simulink model "Control_pendulum_LQR"  (R2023b)
settings: Solver=VariableStepAuto  StartTime=0.0  StopTime=10.0  RelTol=1e-3
settings Model: Creator=Administrator  LastModifiedBy=Administrator

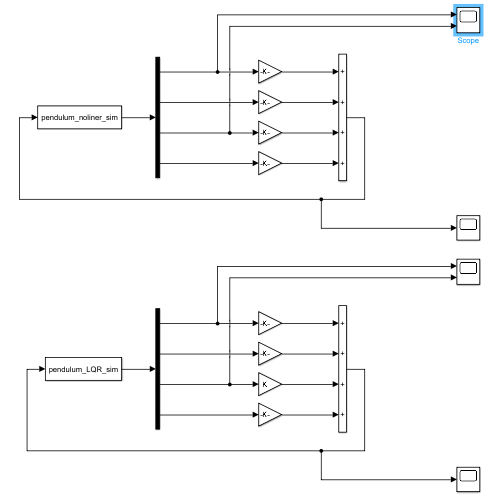
[thumbnail: Simulink's stored preview of the top-level diagram]
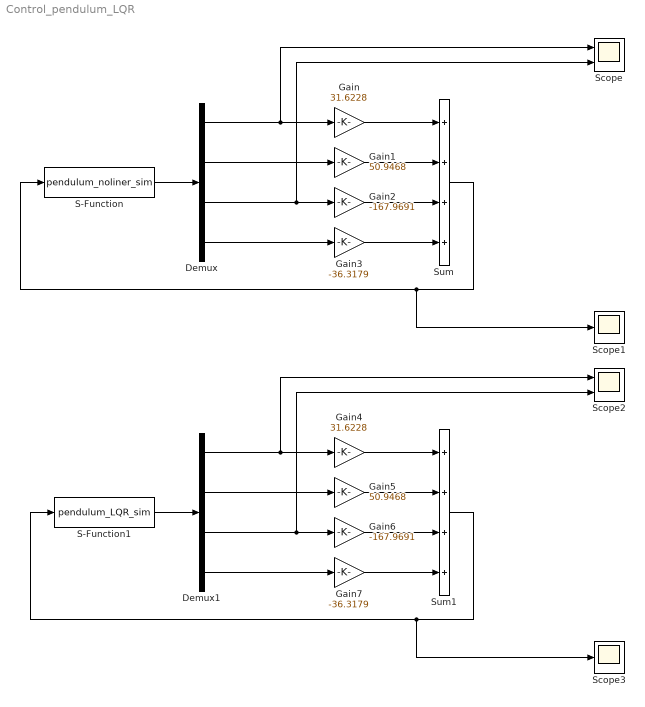
== system Control_pendulum_LQR ==
  Demux : Demux
  Demux1 : Demux
  Gain : Gain  Gain=31.6228
  Gain1 : Gain  Gain=50.9468
  Gain2 : Gain  Gain=-167.9691
  Gain3 : Gain  Gain=-36.3179
  Gain4 : Gain  Gain=31.6228
  Gain5 : Gain  Gain=50.9468
  Gain6 : Gain  Gain=-167.9691
  Gain7 : Gain  Gain=-36.3179
  S-Function : S-Function  FunctionName=pendulum_noliner_sim  SFunctionDeploymentMode=off  EnableBusSupport=off
  S-Function1 : S-Function  FunctionName=pendulum_LQR_sim  SFunctionDeploymentMode=off  EnableBusSupport=off
  Scope : Scope  NumInputPorts=2
  Scope1 : Scope
  Scope2 : Scope  NumInputPorts=2
  Scope3 : Scope
  Sum : Sum  Inputs=++++
  Sum1 : Sum  Inputs=++++
  wires:
  S-Function/1 -> Demux/1
  Demux/1 -> Scope/1, Gain/1
  Demux/4 -> Gain3/1
  Demux/3 -> Scope/2, Gain2/1
  Demux/2 -> Gain1/1
  Gain2/1 -> Sum/3
  Gain3/1 -> Sum/4
  Gain/1 -> Sum/1
  Gain1/1 -> Sum/2
  Sum/1 -> Scope1/1, S-Function/1
  Sum1/1 -> Scope3/1, S-Function1/1
  Demux1/3 -> Scope2/2, Gain6/1
  Demux1/1 -> Scope2/1, Gain4/1
  Gain5/1 -> Sum1/2
  Demux1/2 -> Gain5/1
  Gain7/1 -> Sum1/4
  Gain6/1 -> Sum1/3
  S-Function1/1 -> Demux1/1
  Demux1/4 -> Gain7/1
  Gain4/1 -> Sum1/1
